simulink model "PositionComplementary"  (Simulink 6.6)
settings: Solver=ode4  StartTime=0.0  StopTime=60  FixedStep=SampleT  RelTol=1e-3
InitFcn:
  | clc
  | Taxi_Var_new
  | failures
  | insInit
  | piccolo_init
values from neighbouring files (symbols this model uses):
  A1 = 0    [Taxi_Var.m]    (also in Taxi_Var_new.m = 0.007)
  Apolar = 0.0899    [Taxi_Var.m]    (also in Taxi_Var_new.m = 0.057)
  CD0 = 0.0219    [Taxi_Var.m]    (also in Taxi_Var_new.m = 0.022)
  chord = S/span    (= 0.384036716878)    [Taxi_Var.m]    (also in Taxi_Var_new.m = 0.351341681574)
  CL0 = 0.1857    [Taxi_Var.m]    (also in Taxi_Var_new.m = 0.38)
  CLa = 4.6206    [Taxi_Var.m]    (also in Taxi_Var_new.m = 18.5)
  CLa_dot = 1.93    [Taxi_Var.m]    (also in Taxi_Var_new.m = 2.64)
  Clb = -0.0043    [Taxi_Var.m]    (also in Taxi_Var_new.m = -0.06)
  ClDa = 0.1695    [Taxi_Var.m]    (also in Taxi_Var_new.m)
  CLDe = 0.4032    [Taxi_Var.m]    (also in Taxi_Var_new.m = 0.24)
  CLDf = 0.047    [Taxi_Var.m]    (also in Taxi_Var_new.m = 0.4)
  ClDr = 0.0003    [Taxi_Var.m]    (also in Taxi_Var_new.m = 0.055)
  Clp = -0.4425    [Taxi_Var.m]    (also in Taxi_Var_new.m = -0.88)
  CLq = 8.7465    [Taxi_Var.m]    (also in Taxi_Var_new.m = 7.4)
  Clr = 0.0675    [Taxi_Var.m]    (also in Taxi_Var_new.m = 0.04)
  Cm0 = -0.0902    [Taxi_Var.m]    (also in Taxi_Var_new.m = 0.56)
  Cma = -1.3995    [Taxi_Var.m]    (also in Taxi_Var_new.m = -1.58)
  CmDe = -0.9493    [Taxi_Var.m]    (also in Taxi_Var_new.m = -41)
  CmDf = -.021    (= -0.021)    [Taxi_Var.m]    (also in Taxi_Var_new.m)
  Cmq = -10.8760    (= -10.876)    [Taxi_Var.m]    (also in Taxi_Var_new.m = -12)
  Cnb = 0.0281    [Taxi_Var.m]    (also in Taxi_Var_new.m = 0.73)
  CnDa = -0.0031    [Taxi_Var.m]    (also in Taxi_Var_new.m = -0.032)
  CnDr = -0.0882    [Taxi_Var.m]    (also in Taxi_Var_new.m = 0.19)
  Cnp = -0.0695    [Taxi_Var.m]    (also in Taxi_Var_new.m = -0.1)
  Cnr = -0.1045    [Taxi_Var.m]    (also in Taxi_Var_new.m = -0.23)
  CYb = -0.1999    [Taxi_Var.m]    (also in Taxi_Var_new.m = -0.98)
  CYDr = 0.0192    [Taxi_Var.m]    (also in Taxi_Var_new.m = 0.066)
  damax = 25*deg2rad    (= 0.436332312999)    [Taxi_Var.m]    (also in piccolo_init.m)
  damin = -25*deg2rad    (= -0.436332312999)    [Taxi_Var.m]    (also in piccolo_init.m)
  datrim = 0*deg2rad    (= 0)    [Taxi_Var.m]    (also in piccolo_init.m)
  demax = 15*deg2rad    (= 0.261799387799)    [Taxi_Var.m]    (also in piccolo_init.m)
  demin = -15*deg2rad    (= -0.261799387799)    [Taxi_Var.m]    (also in piccolo_init.m)
  detrim = -2.4137*deg2rad    (= -0.0421270121554)    [Taxi_Var.m]    (also in piccolo_init.m = -0.0523598775598)
  dfland = 30*deg2rad    (= 0.523598775598)    [Taxi_Var.m]    (also in piccolo_init.m)
  dfmax = 30*deg2rad    (= 0.523598775598)    [Taxi_Var.m]    (also in piccolo_init.m)
  dfmin = 0*deg2rad    (= 0)    [Taxi_Var.m]    (also in piccolo_init.m)
  drmax = 25*deg2rad    (= 0.436332312999)    [Taxi_Var.m]    (also in piccolo_init.m)
  drmin = -25*deg2rad    (= -0.436332312999)    [Taxi_Var.m]    (also in piccolo_init.m)
  drtrim = 0*deg2rad    (= 0)    [Taxi_Var.m]    (also in piccolo_init.m)
  dtmax = 1    [Taxi_Var.m]    (also in piccolo_init.m = 0.7)
  dtmin = 0    [Taxi_Var.m]    (also in piccolo_init.m = 0.25)
  dttrim = 0.0725    [Taxi_Var.m]    (also in piccolo_init.m = 0.35)
  Euler_0 = [0; 0; 45]'*pi/180    [Taxi_Var.m]    (also in Taxi_Var_new.m = [0 0 45]'*pi/180)
  IdxCmdOrbitRadius = 17    [piccolo_init.m]
  IdxCmdOrbitSense = 18    [piccolo_init.m]
  IdxCmdWp1Alt = 13    [piccolo_init.m]
  IdxCmdWp1Lat = 11    [piccolo_init.m]
  IdxCmdWp1Lon = 12    [piccolo_init.m]
  IdxCmdWp2Alt = 16    [piccolo_init.m]
  IdxCmdWp2Lat = 14    [piccolo_init.m]
  IdxCmdWp2Lon = 15    [piccolo_init.m]
  IdxEstimReserved1 = 4    [piccolo_init.m]
  IdxEstimWEast = 3    [piccolo_init.m]
  IdxEstimWNorth = 2    [piccolo_init.m]
  IdxGainsAltD = 10    [piccolo_init.m]
  IdxGainsAltI = 9    [piccolo_init.m]
  IdxGainsAltP = 8    [piccolo_init.m]
  IdxGainsPdynD = 4    [piccolo_init.m]
  IdxGainsPdynI = 3    [piccolo_init.m]
  IdxGainsPdynP = 2    [piccolo_init.m]
  IdxGainsPitchD = 7    [piccolo_init.m]
  IdxGainsPitchI = 6    [piccolo_init.m]
  IdxGainsPitchP = 5    [piccolo_init.m]
  IdxGainsRollD = 17    [piccolo_init.m]
  IdxGainsRollI = 16    [piccolo_init.m]
  IdxGainsRollP = 15    [piccolo_init.m]
  IdxGainsSlopeElevatorD = 25    [piccolo_init.m]
  IdxGainsSlopeElevatorP = 26    [piccolo_init.m]
  IdxGainsTrackConv = 24    [piccolo_init.m]
  IdxGainsTrackD = 23    [piccolo_init.m]
  IdxGainsTrackI = 22    [piccolo_init.m]
  IdxGainsTrackP = 21    [piccolo_init.m]
  IdxGainsTurnD = 14    [piccolo_init.m]
  IdxGainsTurnI = 13    [piccolo_init.m]
  IdxGainsTurnP = 12    [piccolo_init.m]
  IdxGainsYawD = 20    [piccolo_init.m]
  IdxGainsYawI = 19    [piccolo_init.m]
  IdxGainsYawP = 18    [piccolo_init.m]
  IdxLimitsAileronMax = 11    [piccolo_init.m]
  IdxLimitsAileronMin = 10    [piccolo_init.m]
  IdxLimitsBankMax = 9    [piccolo_init.m]
  IdxLimitsBankMin = 8    [piccolo_init.m]
  IdxLimitsElevatorMax = 13    [piccolo_init.m]
  IdxLimitsElevatorMin = 12    [piccolo_init.m]
  IdxLimitsFlapMax = 19    [piccolo_init.m]
  IdxLimitsFlapMin = 18    [piccolo_init.m]
  IdxLimitsPdynMax = 3    [piccolo_init.m]
  IdxLimitsPdynMin = 2    [piccolo_init.m]
  IdxLimitsRudderMax = 15    [piccolo_init.m]
  IdxLimitsRudderMin = 14    [piccolo_init.m]
  IdxLimitsThrottleMax = 17    [piccolo_init.m]
  IdxLimitsThrottleMin = 16    [piccolo_init.m]
  IdxSensorsAlt = 5    [piccolo_init.m]
  IdxSensorsLat = 3    [piccolo_init.m]
  IdxSensorsLon = 4    [piccolo_init.m]
  IdxSensorsVDown = 8    [piccolo_init.m]
  IdxSensorsVEast = 7    [piccolo_init.m]
  IdxSensorsVNorth = 6    [piccolo_init.m]
  IdxStatesGlobal = 2    [piccolo_init.m]
  IdxStatesManual = 16    [piccolo_init.m]
  IdxStatesMode = 15    [piccolo_init.m]
  ISA_g = 9.815    [Taxi_Var.m]    (also in Taxi_Var_new.m)
  ISA_hmax = 2000    [Taxi_Var.m]    (also in Taxi_Var_new.m)
  ISA_lapse = .0065    (= 0.0065)    [Taxi_Var.m]    (also in Taxi_Var_new.m)
  ISA_P0 = 101325    [Taxi_Var.m]    (also in Taxi_Var_new.m)
  ISA_R = 287    [Taxi_Var.m]    (also in Taxi_Var_new.m)
  ISA_rho0 = 1.225    [Taxi_Var.m]    (also in Taxi_Var_new.m)
  ISA_T0 = 289    [Taxi_Var.m]    (also in Taxi_Var_new.m)
  Ixx = 3.689084    [Taxi_Var.m]    (also in Taxi_Var_new.m = 3.8)
  Iyy = 7.43789    [Taxi_Var.m]    (also in Taxi_Var_new.m = 9.58)
  Izz = 10.22202    [Taxi_Var.m]    (also in Taxi_Var_new.m = 9.68)
  mass = 22.5    [Taxi_Var.m]    (also in Taxi_Var_new.m = 8.16466266)
  MinThK = 0.075    [Taxi_Var.m]    (also in Taxi_Var_new.m = 0.077)
  Pos_0 = [0; 0; 1000]'    [Taxi_Var.m]    (also in Taxi_Var_new.m = [0 0 500]')
  PQR_0 = [0; 0; 0]'    [Taxi_Var.m]    (also in Taxi_Var_new.m = [ 0 0 0]'*pi/180)
  SampleT = 0.005    [failures.m]
  span = 2.3368    [Taxi_Var.m]    (also in Taxi_Var_new.m = 2.795)
  TFact = 0.4    [Taxi_Var.m]    (also in Taxi_Var_new.m)
  ThK = 2.18    [Taxi_Var.m]    (also in Taxi_Var_new.m = 2.17)
  tsamp = APtsamp    (= 0.05)    [piccolo_init.m]
  ... (+1 more)
undefined symbols (not defined in the file or in its folder): clock, Earth, gaind, polesd, WGS84, zerosd
libraries: piccolo_library x60, simulink x45, aerolibconvert2 x13, dspsigops x5, aerolibasang x5, aerolibatmos2 x2, aerolibtransform2 x2, aerolibnav x2, aerolibutil x1, dspmtrx3 x1
(part 1 of 5)
CloseFcn:
  | rtwprivate ssgencode ModelCloseRequest AttitudeComplementary
settings Model: Creator=ASL_Lab  LastModifiedBy=ASL_Lab
settings DebuggingCC: MultiTaskDSMMsg=warning  MultiTaskCondExecSysMsg=none  StrictBusMsg=None
settings HardwareCC: TargetHWDeviceType=32-bit Generic
settings RTWCC: IncludeERTFirstTime=on

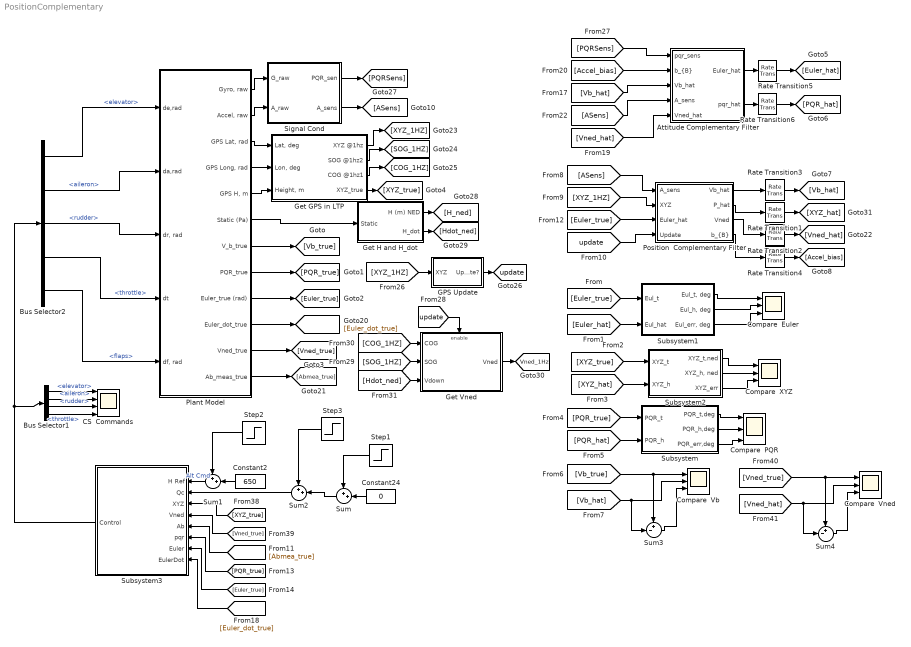
== system PositionComplementary ==
  Attitude Complementary Filter : Subsystem  mask{K1=25, K2=0.1, T=0.01, P0=Euler_0}
      mask prompts: K1 "Euler Gain K1"; K2 "Bias Gain K2"; T "Filter Execution Time"; P0 "Initial Euler"
      mask help: Attitude Complementary filter based on the Magneto-Pendular Sensor by Vasconcelos, et.al.
      mask Help: Help
  Bus Selector1 : BusSelector  OutputSignals=elevator,aileron,rudder,throttle
  Bus Selector2 : BusSelector  OutputSignals=elevator,aileron,rudder,throttle,flaps
  CS  Commands : Scope  NumInputPorts=4
      settings: TimeRange=44  YMin=0.0142~-2.5e-018~-1e-017~0.665  YMax=0.014425~2e-018~1e-017~0.735  SaveName=ScopeData19
  Compare  Euler : Scope  NumInputPorts=3
      settings: TimeRange=60  YMin=-20~-25.33803644914775~-0.3641680926328546  YMax=120~112.0265390106658~0.313830848443414  SaveName=ScopeData20
  Compare  PQR : Scope  NumInputPorts=3
      settings: TimeRange=200  YMin=-50~-350000~-450000  YMax=55~450000~350000  SaveName=ScopeData8
  Compare  Vb : Scope  NumInputPorts=3
      settings: TimeRange=44  YMin=-2.5~-800~-400  YMax=35~400~800  SaveName=ScopeData12
  Compare  Vned : Scope  NumInputPorts=3
      settings: TimeRange=44  YMin=-2.5~-800~-400  YMax=35~400~800  SaveName=ScopeData24
  Compare  XYZ : Scope  NumInputPorts=3
      settings: TimeRange=45  YMin=-800~-200~-32.89473684210498  YMax=800~1200~32.89473684210498  SaveName=ScopeData2
  Constant2 : Constant  Orientation=left  Value=650
  Constant24 : Constant  Orientation=left  Value=0
  GPS Update : Subsystem
  Get GPS in LTP : Subsystem
  "Get H and H_dot " : Subsystem
  Get Vned : Subsystem
  Plant Model : Subsystem
  Position  Complementary Filter : Subsystem  mask{K1=50, K2=75, K3=0.1, T=0.01, P0=Pos_0}
      mask prompts: K1 "Position Gain K1"; K2 "Velocity Gain K2"; K3 "Bias Gain K3"; T "Filter Execution Time"; P0 "Initial Position"
      mask help: Position Complementary filter based on the Magneto-Pendular Sensor by Vasconcelos, et.al.
      mask Help: Help
  Rate Transition{1..6} (6 alike) : RateTransition  OutPortSampleTime=0.005
  Signal Cond : Subsystem
  Step1 : Step  Orientation=left  Time=15  After=3*pi/180  SampleTime=0
  Step2 : Step  Orientation=left  Time=35  After=250  SampleTime=0
  Step3 : Step  Orientation=left  Time=35  After=-4*pi/180  SampleTime=0
  Subsystem : Subsystem
  Subsystem1 : Subsystem
  Subsystem2 : Subsystem
  Subsystem3 : Subsystem  Orientation=left
  Sum : Sum  Orientation=left  Inputs=++|  SaturateOnIntegerOverflow=on
  Sum1 : Sum  Orientation=left  Inputs=++|  SaturateOnIntegerOverflow=on
  Sum2 : Sum  Orientation=left  Inputs=++|  SaturateOnIntegerOverflow=on
  Sum3 : Sum  Inputs=+-|
  Sum4 : Sum  Inputs=+-|
  tag scope: Vned_1Hz=global, update=global
  wires:
  Plant Model/1("Gyro, raw") -> Signal Cond/1(G_raw)
  Plant Model/2("Accel, raw") -> Signal Cond/2(A_raw)
  Plant Model/3("GPS Lat, rad") -> Get GPS in LTP/1("Lat, deg")
  Plant Model/5("GPS H, m") -> Get GPS in LTP/3("Height, m")
  Plant Model/4("GPS Long, rad") -> Get GPS in LTP/2("Lon, deg")
  Plant Model/7(V_b_true) -> [Vb_true]
  Plant Model/8(PQR_true) -> [PQR_true]
  Plant Model/9(Euler_true (rad)) -> [Euler_true]
  Plant Model/11(Vned_true) -> [Vned_true]
  Subsystem1/1("Eul_t, deg") -> Compare  Euler/1
  Subsystem1/2("Eul_h, deg") -> Compare  Euler/2
  Subsystem1/3("Eul_err, deg") -> Compare  Euler/3
  [XYZ_true] -> Subsystem2/1(XYZ_t)
  [XYZ_hat] -> Subsystem2/2(XYZ_h)
  Subsystem/1(PQR_t,deg) -> Compare  PQR/1
  Subsystem/2(PQR_h,deg) -> Compare  PQR/2
  Subsystem/3(PQR_err,deg) -> Compare  PQR/3
  [Vb_true] -> Compare  Vb/1, Sum3/1
  [Vb_hat] -> Sum3/2, Compare  Vb/2
  Sum3/1 -> Compare  Vb/3
  Get GPS in LTP/4(XYZ_true) -> [XYZ_true]
  [PQR_true] -> Subsystem/1(PQR_t)
  [PQR_hat] -> Subsystem/2(PQR_h)
  [Euler_true] -> Subsystem1/1(Eul_t)
  [Euler_hat] -> Subsystem1/2(Eul_hat)
  Subsystem2/1(XYZ_t,ned) -> Compare  XYZ/1
  Subsystem2/2("XYZ_h, ned") -> Compare  XYZ/2
  Subsystem2/3(XYZ_err) -> Compare  XYZ/3
  Constant24/1 -> Sum/2
  Step1/1 -> Sum/1
  Constant2/1 -> Sum1/2
  Step2/1 -> Sum1/1
  Plant Model/10(Euler_dot_true) -> [Euler_dot_true]
  Plant Model/12(Ab_meas_true) -> [Abmea_true]
  Plant Model/6(Static (Pa)) -> "Get H and H_dot "/1(Static)
  Signal Cond/2(A_sens) -> [ASens]
  Get GPS in LTP/1(XYZ @1hz) -> [XYZ_1HZ]
  Get GPS in LTP/2(SOG @1hz2) -> [SOG_1HZ]
  Get GPS in LTP/3(COG @1hz1) -> [COG_1HZ]
  GPS Update/1(Update?) -> [update]
  [XYZ_1HZ] -> GPS Update/1(XYZ)
  Signal Cond/1(PQR_sen) -> [PQRSens]
  [update] -> Get Vned/Enable
  [COG_1HZ] -> Get Vned/1(COG)
  [SOG_1HZ] -> Get Vned/2(SOG)
  "Get H and H_dot "/1(H (m) NED) -> [H_ned]
  "Get H and H_dot "/2(H_dot) -> [Hdot_ned]
  [Hdot_ned] -> Get Vned/3(Vdown)
  Get Vned/1(Vned) -> [Vned_1Hz]
  Sum1/1 -> Subsystem3/1(H Ref)  "Alt Cmd"
  [ASens] -> Position  Complementary Filter/1(A_sens)
  [XYZ_1HZ] -> Position  Complementary Filter/2(XYZ)
  [Euler_true] -> Position  Complementary Filter/3(Euler_hat)
  [update] -> Position  Complementary Filter/4(Update)
  Position  Complementary Filter/1(Vb_hat) -> Rate Transition3/1
  Position  Complementary Filter/2(P_hat) -> Rate Transition1/1
  [XYZ_true] -> Subsystem3/3(XYZ)
  [Vned_true] -> Subsystem3/4(Vned)
  [Abmea_true] -> Subsystem3/5(Ab)
  [PQR_true] -> Subsystem3/6(pqr)
  [Euler_true] -> Subsystem3/7(Euler)
  [Euler_dot_true] -> Subsystem3/8(EulerDot)
  Subsystem3/1(Control) -> Bus Selector2/1, Bus Selector1/1
  Bus Selector2/1 -> Plant Model/1(de,rad)  "<elevator>"
  Bus Selector2/2 -> Plant Model/2(da,rad)  "<aileron>"
  Bus Selector2/3 -> Plant Model/3("dr, rad")  "<rudder>"
  Bus Selector2/4 -> Plant Model/4(dt)  "<throttle>"
  Bus Selector2/5 -> Plant Model/5("df, rad")  "<flaps>"
  Rate Transition3/1 -> [Vb_hat]
  Rate Transition1/1 -> [XYZ_hat]
  Bus Selector1/1 -> CS  Commands/1  "<elevator>"
  Bus Selector1/2 -> CS  Commands/2  "<aileron>"
  Bus Selector1/3 -> CS  Commands/3  "<rudder>"
  Bus Selector1/4 -> CS  Commands/4  "<throttle>"
  Sum2/1 -> Subsystem3/2(Qc)
  Sum/1 -> Sum2/2
  Step3/1 -> Sum2/1
  Rate Transition2/1 -> [Vned_hat]
  Position  Complementary Filter/3(Vned) -> Rate Transition2/1
  [Vned_true] -> Sum4/1, Compare  Vned/1
  [Vned_hat] -> Compare  Vned/2, Sum4/2
  Sum4/1 -> Compare  Vned/3
  Position  Complementary Filter/4("b_{B}") -> Rate Transition4/1
  Rate Transition4/1 -> [Accel_bias]
  [PQRSens] -> Attitude Complementary Filter/1(pqr_sens)
  Attitude Complementary Filter/1(Euler_hat) -> Rate Transition5/1
  Attitude Complementary Filter/2(pqr_hat) -> Rate Transition6/1
  [ASens] -> Attitude Complementary Filter/4(A_sens)
  [Accel_bias] -> Attitude Complementary Filter/2("b_{B}")
  [Vb_hat] -> Attitude Complementary Filter/3(Vb_hat)
  [Vned_hat] -> Attitude Complementary Filter/5(Vned_hat)
  Rate Transition5/1 -> [Euler_hat]
  Rate Transition6/1 -> [PQR_hat]

== system PositionComplementary/Attitude Complementary Filter ==
  pqr_sens : Inport
  "b_{B}" : Inport  Port=2
  Vb_hat : Inport  Port=3
  A_sens : Inport  Port=4
  Vned_hat : Inport  Port=5
  Embedded MATLAB Function : Stateflow chart
  Embedded MATLAB Function1 : Stateflow chart
  IC : InitialCondition  Value=P0  SampleTime=T
  Integer Delay4 : simulink/Discrete/Integer Delay  Orientation=left  vinit=0.0  samptime=-1  NumDelays=1
  Integer Delay5 : simulink/Discrete/Integer Delay  Orientation=left  vinit=0.0  samptime=-1  NumDelays=1
  K1 : Gain  Orientation=left  Gain=K1
  K2 : Gain  Orientation=left  Gain=K2
  Subsystem : Subsystem
  Sum5 : Sum  Orientation=down  Inputs=-+|
  Sum6 : Sum  Inputs=|++
  Sum8 : Sum  Inputs=4
  T3 : Gain  Gain=T
  T4 : Gain  Gain=T
  inertial to body : Stateflow chart
  Euler_hat : Outport  Orientation=left
  pqr_hat : Outport  Orientation=left  Port=2
  wires:
  Embedded MATLAB Function/1(euler_dot) -> T3/1
  Subsystem/1(Euler) -> [Euler], Embedded MATLAB Function/1(euler)
  T3/1 -> Sum8/1
  Subsystem/2(pqr_nb) -> Embedded MATLAB Function/2(pqr), pqr_hat/1
  Sum8/1 -> Integer Delay4/1, Euler_hat/1, IC/1
  [Euler] -> Sum5/2
  Integer Delay4/1 -> Sum8/4
  K1/1 -> Sum8/3
  inertial to body/1(pqr) -> Sum6/1
  Sum6/1 -> Embedded MATLAB Function1/2(pqr), Integer Delay5/1, [bg_b]
  [Euler] -> Embedded MATLAB Function1/1(euler)
  [Euler] -> inertial to body/1(euler)
  Embedded MATLAB Function1/1(euler_dot) -> T4/1
  T4/1 -> Sum8/2
  Integer Delay5/1 -> Sum6/2
  K2/1 -> inertial to body/2(euler_dot)
  [bg_b] -> Subsystem/1("bg_{B}")
  pqr_sens/1 -> Subsystem/2(pqr_sens)
  "b_{B}"/1 -> Subsystem/3("b_{B}")
  Vb_hat/1 -> Subsystem/4(Vb_hat)
  A_sens/1 -> Subsystem/5(A_sens)
  Vned_hat/1 -> Subsystem/6(Vned_hat)
  Sum5/1 -> K1/1, K2/1
  IC/1 -> Sum5/1

== system PositionComplementary/GPS Update ==
  XYZ : Inport
  Demux : Demux  Outputs=3
  Detect Change : Subsystem
  Detect Change1 : Subsystem
  Detect Change2 : Subsystem
  Saturation1 : Saturate  UpperLimit=1  LowerLimit=0  SampleTime=SampleT
  Sum : Sum  Inputs=3
  Update? : Outport
  wires:
  Demux/1 -> Detect Change/1(Data)
  Demux/2 -> Detect Change1/1(Data)
  Demux/3 -> Detect Change2/1(Data)
  Detect Change/1(change?) -> Sum/1
  Detect Change1/1(change?) -> Sum/2
  Detect Change2/1(change?) -> Sum/3
  Sum/1 -> Saturation1/1
  XYZ/1 -> Demux/1
  Saturation1/1 -> Update?/1

== system PositionComplementary/Get GPS in LTP ==
  "Lat, deg" : Inport
  "Lon, deg" : Inport  Port=2
  "Height, m" : Inport  Port=3
  Angle Conversion1 : aerolibconvert2/Angle Conversion  SystemSampleTime=-1  IU=rad  OU=deg
  Angle Conversion2 : aerolibconvert2/Angle Conversion  SystemSampleTime=-1  IU=rad  OU=deg
  Constant : Constant  Orientation=left  Value=[0 , 37.0004768371582, -122.061897277832]
  Demux : Demux  Outputs=3
  Demux1 : Demux  Outputs=3
  Discrete Derivative : simulink/Discrete/Discrete Derivative  SystemSampleTime=-1  gainval=1.0  ICPrevScaledInput=0.0  OutDataType=sfix(16)  OutScaling=2^-10  DoSatur=off
  Embedded MATLAB Function1 : Stateflow chart
  Fcn : Fcn  Expr=sqrt(u(1)^2+u(2)^2+u(3)^2)
  Geod2LTP2 : Subsystem
      mask Description:
      | This block provides transformation of the Geodetic coordinates
      | to the LTP coorinate system. The block uses two consecutive transformations
      | (Geodetic -> ECEF ->LTP).
      | Geodetic coordinates of the LTP origin should also be predetermined.
      mask Help: Oops!
      mask Display: plot(0,0,100,100,[45,40,35,40,40],[85,95,85,95,40],[85,95,85,95,40],[35,40,45,40,40],[60,40,10,20,10,14],[70,40,10,13,10,20],[56,45],[70,70],[60,60],[50,60],[60,60],[30,40],[50,60],[20,20],[30,40],[20,20],[45,55],[35,25],[75,65],[35,25])
  Mux : Mux  Inputs=3
  NEU2NED : Gain  Gain=[1 0 0;0 1 0;0 0 -1]  Multiplication=Matrix(K*u)  SaturateOnIntegerOverflow=on
  NEU2NED1 : Gain  Gain=[1 0 0;0 1 0;0 0 -1]  Multiplication=Matrix(K*u)  SaturateOnIntegerOverflow=on
  Reshape1 : Reshape
  Sim Latency : Subsystem
  Sim Latency3 : Subsystem
  Sim Latency4 : Subsystem
  Sim Latency5 : Subsystem
  Sim Latency6 : Subsystem
  XYZ @1hz : Outport
  SOG @1hz2 : Outport  Port=2
  COG @1hz1 : Outport  Port=3
  XYZ_true : Outport  Port=4
  wires:
  Constant/1 -> Geod2LTP2/1("Height, Lat, Lon Initials from GPS")
  Geod2LTP2/1("NEU, m") -> Demux1/1, Discrete Derivative/1, Reshape1/1
  "Lat, deg"/1 -> Angle Conversion1/1
  "Lon, deg"/1 -> Angle Conversion2/1
  "Height, m"/1 -> Geod2LTP2/4(Hight,m(GPS))
  Fcn/1 -> Sim Latency6/1(Fast Data)
  Embedded MATLAB Function1/1(cog) -> Sim Latency5/1(Fast Data)
  Discrete Derivative/1 -> Demux/1, Fcn/1
  Mux/1 -> NEU2NED1/1
  Angle Conversion1/1 -> Geod2LTP2/2("Lat, deg(GPS)")
  Angle Conversion2/1 -> Geod2LTP2/3("Lon, deg(GPS)")
  Demux1/1 -> Sim Latency/1(Fast Data)
  Demux1/2 -> Sim Latency3/1(Fast Data)
  Demux1/3 -> Sim Latency4/1(Fast Data)
  Sim Latency/1(1Hz Data) -> Mux/1
  Sim Latency3/1(1Hz Data) -> Mux/2
  Sim Latency4/1(1Hz Data) -> Mux/3
  Sim Latency5/1(1Hz Data) -> COG @1hz1/1
  Sim Latency6/1(1Hz Data) -> SOG @1hz2/1
  Reshape1/1 -> NEU2NED/1
  NEU2NED/1 -> XYZ_true/1
  Demux/1 -> Embedded MATLAB Function1/1(Vn)
  Demux/2 -> Embedded MATLAB Function1/2(Ve)
  NEU2NED1/1 -> XYZ @1hz/1

== system PositionComplementary/Get H and H_dot  ==
  Static : Inport
  Discrete Derivative : simulink/Discrete/Discrete Derivative  SystemSampleTime=-1  gainval=1.0  ICPrevScaledInput=-0.6  OutDataType=sfix(16)  OutScaling=2^-10  DoSatur=off
  Gain : Gain  Gain=-1
  Pressure Altitude : aerolibatmos2/Pressure Altitude  SystemSampleTime=-1  units=Metric (MKS)  action=Warning
  H (m) NED : Outport
  H_dot : Outport  Port=2
  wires:
  Pressure Altitude/1 -> Gain/1
  Gain/1 -> Discrete Derivative/1, H (m) NED/1
  Discrete Derivative/1 -> H_dot/1
  Static/1 -> Pressure Altitude/1

== system PositionComplementary/Get Vned ==
  COG : Inport
  SOG : Inport  Port=2
  Vdown : Inport  Port=3
  Enable : EnablePort
  Embedded MATLAB Function1 : Stateflow chart
  Mux1 : Mux  Inputs=3
  Vned : Outport
  wires:
  Embedded MATLAB Function1/1(Vn) -> Mux1/1
  Embedded MATLAB Function1/2(Ve) -> Mux1/2
  Vdown/1 -> Mux1/3
  Mux1/1 -> Vned/1
  COG/1 -> Embedded MATLAB Function1/2(cog)
  SOG/1 -> Embedded MATLAB Function1/1(sog)

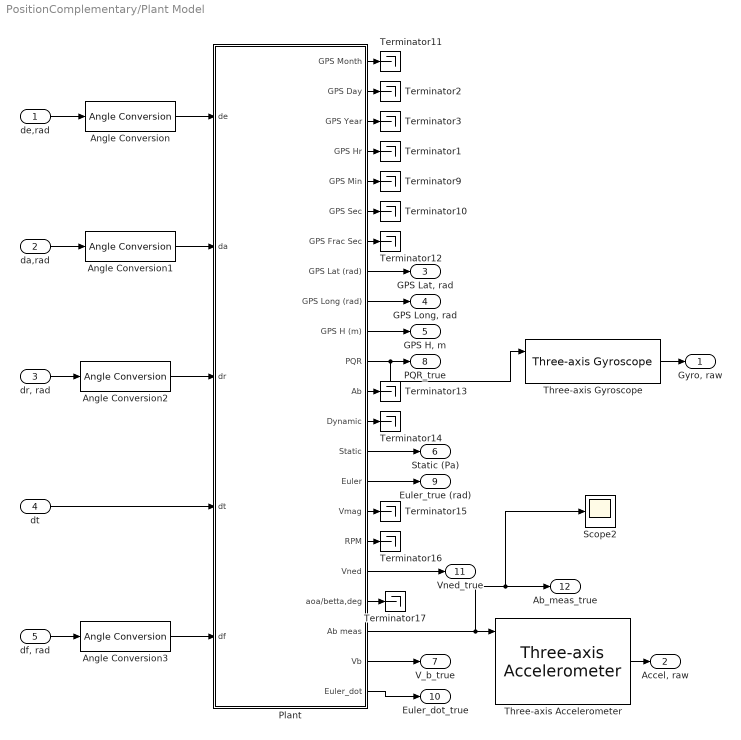
== system PositionComplementary/Plant Model ==
  de,rad : Inport
  da,rad : Inport  Port=2
  "dr, rad" : Inport  Port=3
  dt : Inport  Port=4
  "df, rad" : Inport  Port=5
  Angle Conversion{,1..3} (4 alike) : aerolibconvert2/Angle Conversion  SystemSampleTime=-1  IU=rad  OU=deg
  Plant : Subsystem
  Scope2 : Scope
      settings: TimeRange=44  YMin=-45  YMax=20  SaveName=ScopeData33
  Terminator{1..3,9..17} (12 alike) : Terminator
  Three-axis Accelerometer : aerolibnav/Three-axis Accelerometer  SystemSampleTime=-1  units=Metric (MKS)  acc=[0 0 0]  gtype=off  dtype_a=on  w_a=190  z_a=0.707  a_sf_cc=[-41 0 0; 0 41 0; 0 0 -43]  a_bias=[2015 2018 2006]  a_rand=on  a_seeds=[23093 23094 23095]  a_pow=[0.008 0.008 0.008]  a_sat="[-inf  -inf  -inf  inf inf inf]"  a_Ts=SampleT
  Three-axis Gyroscope : aerolibnav/Three-axis Gyroscope  SystemSampleTime=-1  dtype_g=on  w_g=190  z_g=0.707  g_sf_cc=[-142 0 0; 0 142 0; 0 0 235]  g_bias=[1866 1981 2042]  g_sen=[0 0 0]  g_rand=on  g_seeds=[23093 23094 23095]  g_pow=[0.008 0.008 0.008]  g_sat="[-inf  -inf  -inf  inf inf inf]"  g_Ts=SampleT
  "Gyro, raw" : Outport
  "Accel, raw" : Outport  Port=2
  "GPS Lat, rad" : Outport  Port=3
  "GPS Long, rad" : Outport  Port=4
  "GPS H, m" : Outport  Port=5
  Static (Pa) : Outport  Port=6
  V_b_true : Outport  Port=7
  PQR_true : Outport  Port=8
  Euler_true (rad) : Outport  Port=9
  Euler_dot_true : Outport  Port=10
  Vned_true : Outport  Port=11
  Ab_meas_true : Outport  Port=12
  wires:
  Three-axis Gyroscope/1 -> "Gyro, raw"/1
  Three-axis Accelerometer/1 -> "Accel, raw"/1
  Plant/11(PQR) -> PQR_true/1, Three-axis Gyroscope/1
  Plant/14(Static) -> Static (Pa)/1
  Plant/8(GPS Lat (rad)) -> "GPS Lat, rad"/1
  Plant/9(GPS Long (rad)) -> "GPS Long, rad"/1
  Plant/10(GPS H (m)) -> "GPS H, m"/1
  Plant/20(Ab meas) -> Three-axis Accelerometer/1, Ab_meas_true/1, Scope2/1
  Plant/21(Vb) -> V_b_true/1
  Plant/15(Euler) -> Euler_true (rad)/1
  Plant/18(Vned) -> Vned_true/1
  Plant/1(GPS Month) -> Terminator11/1
  Plant/2(GPS Day) -> Terminator2/1
  Plant/3(GPS Year) -> Terminator3/1
  Plant/4(GPS Hr) -> Terminator1/1
  Plant/5(GPS Min) -> Terminator9/1
  Plant/6(GPS Sec) -> Terminator10/1
  Plant/7(GPS Frac Sec) -> Terminator12/1
  Plant/12(Ab) -> Terminator13/1
  Plant/13(Dynamic) -> Terminator14/1
  Plant/16(Vmag) -> Terminator15/1
  Plant/17(RPM) -> Terminator16/1
  Plant/19(aoa/betta,deg) -> Terminator17/1
  de,rad/1 -> Angle Conversion/1
  da,rad/1 -> Angle Conversion1/1
  "dr, rad"/1 -> Angle Conversion2/1
  dt/1 -> Plant/4(dt)
  "df, rad"/1 -> Angle Conversion3/1
  Angle Conversion/1 -> Plant/1(de)
  Angle Conversion1/1 -> Plant/2(da)
  Angle Conversion2/1 -> Plant/3(dr)
  Angle Conversion3/1 -> Plant/5(df)
  Plant/22(Euler_dot) -> Euler_dot_true/1

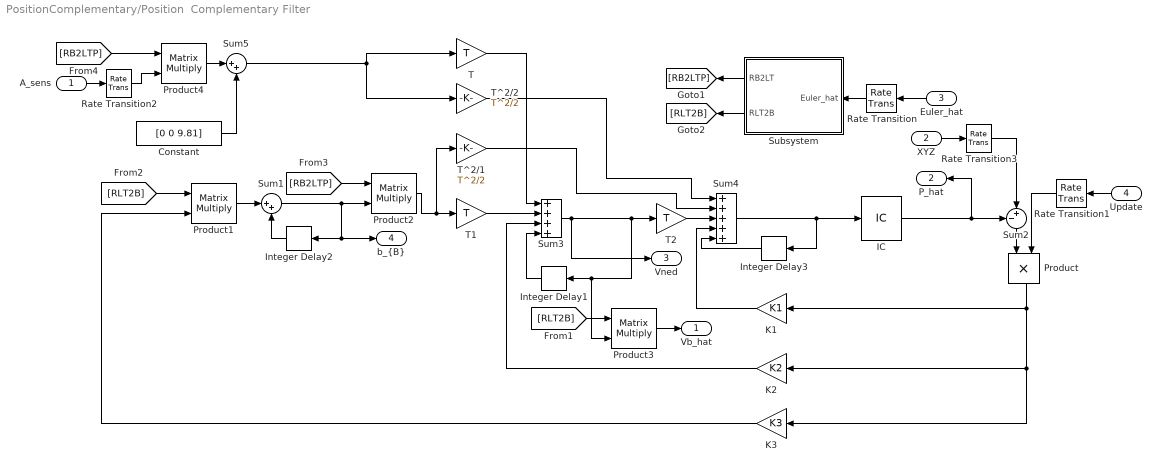
== system PositionComplementary/Position  Complementary Filter ==
  A_sens : Inport
  XYZ : Inport  Port=2
  Euler_hat : Inport  Orientation=left  Port=3
  Update : Inport  Orientation=left  Port=4
  Constant : Constant  Value=[0 0 9.81]  SampleTime=0.01
  IC : InitialCondition  Value=P0  SampleTime=T
  Integer Delay1 : simulink/Discrete/Integer Delay  Orientation=left  vinit=0.0  samptime=-1  NumDelays=1
  Integer Delay2 : simulink/Discrete/Integer Delay  Orientation=left  vinit=0.0  samptime=-1  NumDelays=1
  Integer Delay3 : simulink/Discrete/Integer Delay  Orientation=left  vinit=0.0  samptime=-1  NumDelays=1
  K1 : Gain  Orientation=left  Gain=K1
  K2 : Gain  Orientation=left  Gain=K2
  K3 : Gain  Orientation=left  Gain=K3
  Product : Product  Orientation=down  RndMeth=Zero
  Product{1..4} (4 alike) : Product  Multiplication=Matrix(*)  RndMeth=Zero
  Rate Transition : RateTransition  Orientation=left  OutPortSampleTime=T
  Rate Transition1 : RateTransition  Orientation=left  OutPortSampleTime=T
  Rate Transition2 : RateTransition  OutPortSampleTime=T
  Rate Transition3 : RateTransition  OutPortSampleTime=T
  Subsystem : Subsystem  Orientation=left
  Sum1 : Sum  Inputs=|++
  Sum2 : Sum  Orientation=down  Inputs=-+|
  Sum3 : Sum  Inputs=4
  Sum4 : Sum  Inputs=5
  Sum5 : Sum  Inputs=|++
  T : Gain  Gain=T
  T1 : Gain  Gain=T
  T2 : Gain  Gain=T
  T^2/1 : Gain  Gain=T^2/2
  T^2/2 : Gain  Gain=T^2/2
  Vb_hat : Outport
  P_hat : Outport  Orientation=left  Port=2
  Vned : Outport  Port=3
  "b_{B}" : Outport  Port=4
  wires:
  Subsystem/2(RLT2B) -> [RLT2B]
  Subsystem/1(RB2LT) -> [RB2LTP]
  Euler_hat/1 -> Rate Transition/1
  K3/1 -> Product1/2
  Product1/1 -> Sum1/1
  Sum1/1 -> Product2/2, Integer Delay2/1, "b_{B}"/1
  Product2/1 -> T^2/1/1, T1/1
  T1/1 -> Sum3/2
  T/1 -> Sum3/1
  Sum3/1 -> T2/1, Integer Delay1/1, Product3/2, Vned/1
  K2/1 -> Sum3/3
  T2/1 -> Sum4/3
  T^2/1/1 -> Sum4/2
  T^2/2/1 -> Sum4/1
  Sum4/1 -> Integer Delay3/1, IC/1
  K1/1 -> Sum4/4
  XYZ/1 -> Rate Transition3/1
  Product3/1 -> Vb_hat/1
  Sum2/1 -> Product/1
  Product/1 -> K1/1, K2/1, K3/1
  Update/1 -> Rate Transition1/1
  Integer Delay3/1 -> Sum4/5
  Integer Delay2/1 -> Sum1/2
  Integer Delay1/1 -> Sum3/4
  A_sens/1 -> Rate Transition2/1
  Product4/1 -> Sum5/1
  Constant/1 -> Sum5/2
  Sum5/1 -> T/1, T^2/2/1
  Rate Transition/1 -> Subsystem/1(Euler_hat)
  Rate Transition1/1 -> Product/2
  Rate Transition3/1 -> Sum2/2
  [RLT2B] -> Product1/1
  [RB2LTP] -> Product4/1
  Rate Transition2/1 -> Product4/2
  [RB2LTP] -> Product2/1
  [RLT2B] -> Product3/1
  IC/1 -> Sum2/1, P_hat/1

== system PositionComplementary/Signal Cond ==
  G_raw : Inport
  A_raw : Inport  Port=2
  Accel Convert : Subsystem
  Gyro Convert : Subsystem
  PQR_sen : Outport
  A_sens : Outport  Port=2
  wires:
  G_raw/1 -> Gyro Convert/1(Raw)
  Gyro Convert/1(Comp) -> PQR_sen/1
  A_raw/1 -> Accel Convert/1(Raw)
  Accel Convert/1(Comp) -> A_sens/1

== system PositionComplementary/Subsystem ==
  PQR_t : Inport
  PQR_h : Inport  Port=2
  Angle Conversion1 : aerolibconvert2/Angle Conversion  SystemSampleTime=-1  IU=rad  OU=deg
  Angle Conversion5 : aerolibconvert2/Angle Conversion  SystemSampleTime=-1  IU=rad  OU=deg
  Angle Conversion6 : aerolibconvert2/Angle Conversion  SystemSampleTime=-1  IU=rad  OU=deg
  Sum2 : Sum  Inputs=+-|
  PQR_t,deg : Outport
  PQR_h,deg : Outport  Port=2
  PQR_err,deg : Outport  Port=3
  wires:
  PQR_t/1 -> Angle Conversion6/1, Sum2/1
  PQR_h/1 -> Angle Conversion1/1, Sum2/2
  Sum2/1 -> Angle Conversion5/1
  Angle Conversion6/1 -> PQR_t,deg/1
  Angle Conversion1/1 -> PQR_h,deg/1
  Angle Conversion5/1 -> PQR_err,deg/1

== system PositionComplementary/Subsystem1 ==
  Eul_t : Inport
  Eul_hat : Inport  Port=2
  Angle Conversion2 : aerolibconvert2/Angle Conversion  SystemSampleTime=-1  IU=rad  OU=deg
  Angle Conversion3 : aerolibconvert2/Angle Conversion  SystemSampleTime=-1  IU=rad  OU=deg
  Angle Conversion4 : aerolibconvert2/Angle Conversion  SystemSampleTime=-1  IU=rad  OU=deg
  Sum : Sum  Inputs=+-|
  "Eul_t, deg" : Outport
  "Eul_h, deg" : Outport  Port=2
  "Eul_err, deg" : Outport  Port=3
  wires:
  Eul_t/1 -> Sum/1, Angle Conversion4/1
  Eul_hat/1 -> Sum/2, Angle Conversion2/1
  Sum/1 -> Angle Conversion3/1
  Angle Conversion4/1 -> "Eul_t, deg"/1
  Angle Conversion2/1 -> "Eul_h, deg"/1
  Angle Conversion3/1 -> "Eul_err, deg"/1

== system PositionComplementary/Subsystem2 ==
  XYZ_t : Inport
  XYZ_h : Inport  Port=2
  Sum1 : Sum  Inputs=+-|
  XYZ_t,ned : Outport
  "XYZ_h, ned" : Outport  Port=2
  XYZ_err : Outport  Port=3
  wires:
  XYZ_h/1 -> Sum1/2, "XYZ_h, ned"/1
  XYZ_t/1 -> Sum1/1, XYZ_t,ned/1
  Sum1/1 -> XYZ_err/1

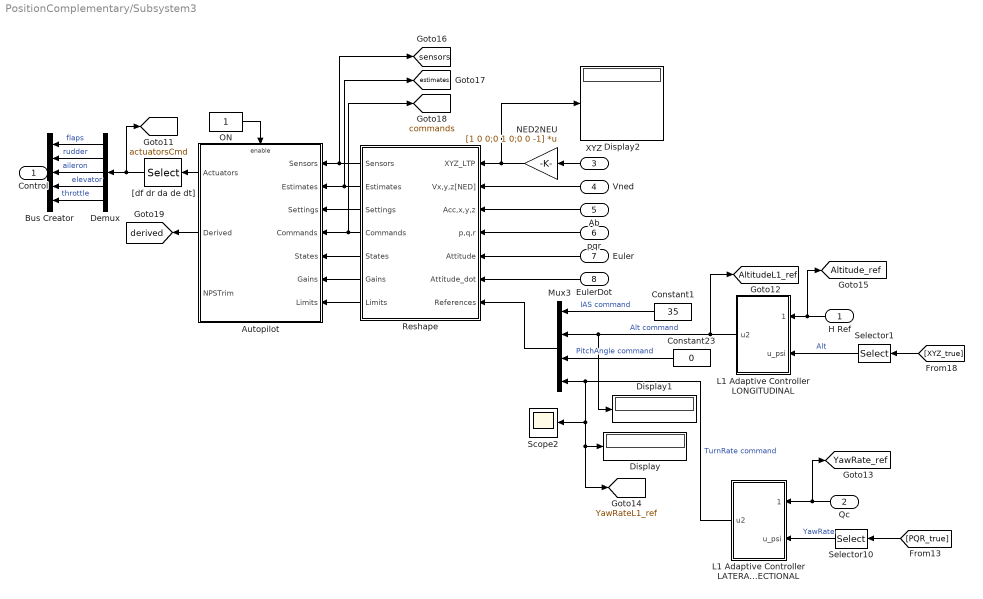
== system PositionComplementary/Subsystem3 ==
  H Ref : Inport  Orientation=left
  Qc : Inport  Orientation=left  Port=2
  XYZ : Inport  Orientation=left  Port=3
  Vned : Inport  Orientation=left  Port=4
  Ab : Inport  Orientation=left  Port=5
  pqr : Inport  Orientation=left  Port=6
  Euler : Inport  Orientation=left  Port=7
  EulerDot : Inport  Orientation=left  Port=8
  Autopilot : Subsystem  Orientation=left
  Bus Creator : BusCreator  Orientation=left  Inputs=5
  Constant1 : Constant  Orientation=left  Value=35
  Constant23 : Constant  Orientation=left  Value=0
  Demux : Demux  Orientation=left  Outputs=5
  Display : Display
  Display1 : Display
  Display2 : Display
  L1 Adaptive Controller LATERAL-DIRECTIONAL : Subsystem  Orientation=left  mask{gamma=-2000, m=4, omega=2, Pbound=.1, L1ONOFF=0}
      mask prompts: gamma "L1 gain"; m "state predictor (m)"; omega "low-pass filter (omega)"; Pbound "projection bounds"; L1ONOFF "L1 switch"
  L1 Adaptive Controller LONGITUDINAL : Subsystem  Orientation=left  mask{gamma=-1, m=4, omega=1, Pbound=50, L1ONOFF=0}
      mask prompts: gamma "L1 gain"; m "state predictor (m)"; omega "low-pass filter (omega)"; Pbound "projection bounds"; L1ONOFF "L1 switch"
  Mux3 : Mux  Orientation=left
  NED2NEU : Gain  Orientation=left  Gain=[1 0 0;0 1 0;0 0 -1]  Multiplication=Matrix(K*u)  SaturateOnIntegerOverflow=on
  ON : Constant
  Reshape : Subsystem  Orientation=left
  Scope2 : Scope
      settings: YMin=-1  YMax=1  SaveName=ScopeData29
  Selector1 : Selector  Orientation=left  IndexOptions=Index vector (dialog)  Indices=3  OutputSizes=1  InputPortWidth=3
  Selector10 : Selector  Orientation=left  IndexOptions=Index vector (dialog)  Indices=3  OutputSizes=1  InputPortWidth=3
  "[df dr da de dt]" : Selector  Orientation=left  IndexOptions=Index vector (dialog)  Indices=[10 6 2 4 8]  OutputSizes=[(-2)]  InputPortWidth=12
  Control : Outport  Orientation=left
  tag scope: AltitudeL1_ref=global, Altitude_ref=global, YawRateL1_ref=global, YawRate_ref=global, actuatorsCmd=global, commands=global, derived=global, estimates=global, sensors=global
  wires:
  XYZ/1 -> NED2NEU/1
  Vned/1 -> Reshape/2(Vx,y,z[NED])
  Ab/1 -> Reshape/3(Acc,x,y,z)
  pqr/1 -> Reshape/4(p,q,r)
  Reshape/1(Sensors) -> Autopilot/1(Sensors), [sensors]
  Reshape/2(Estimates) -> Autopilot/2(Estimates), [estimates]
  Reshape/3(Settings) -> Autopilot/3(Settings)
  Reshape/4(Commands) -> Autopilot/4(Commands), [commands]
  Reshape/5(States) -> Autopilot/5(States)
  Reshape/6(Gains) -> Autopilot/6(Gains)
  Reshape/7(Limits) -> Autopilot/7(Limits)
  ON/1 -> Autopilot/Enable
  Autopilot/1(Actuators) -> "[df dr da de dt]"/1
  "[df dr da de dt]"/1 -> Demux/1, [actuatorsCmd]
  Euler/1 -> Reshape/5(Attitude)
  EulerDot/1 -> Reshape/6(Attitude_dot)
  Autopilot/2(Derived) -> [derived]
  Constant1/1 -> Mux3/1  "IAS command"
  L1 Adaptive Controller LONGITUDINAL/1(u2) -> [AltitudeL1_ref], Mux3/2, Display1/1  "Alt command"
  Constant23/1 -> Mux3/3  "PitchAngle command"
  L1 Adaptive Controller LATERAL-DIRECTIONAL/1(u2) -> Mux3/4, Display/1, [YawRateL1_ref], Scope2/1  "TurnRate command"
  Mux3/1 -> Reshape/7(References)
  Qc/1 -> L1 Adaptive Controller LATERAL-DIRECTIONAL/1(u_psi_c), [YawRate_ref]
  [PQR_true] -> Selector10/1
  Selector10/1 -> L1 Adaptive Controller LATERAL-DIRECTIONAL/2(u_psi)  "YawRate"
  H Ref/1 -> L1 Adaptive Controller LONGITUDINAL/1(u_psi_c), [Altitude_ref]
  [XYZ_true] -> Selector1/1
  Selector1/1 -> L1 Adaptive Controller LONGITUDINAL/2(u_psi)  "Alt"
  Demux/1 -> Bus Creator/1  "flaps"
  Demux/2 -> Bus Creator/2  "rudder"
  Demux/3 -> Bus Creator/3  "aileron"
  Demux/4 -> Bus Creator/4  "elevator"
  Demux/5 -> Bus Creator/5  "throttle"
  NED2NEU/1 -> Reshape/1(XYZ_LTP), Display2/1
  Bus Creator/1 -> Control/1

== system PositionComplementary/Attitude Complementary Filter/Subsystem ==
  "bg_{B}" : Inport  Orientation=left
  pqr_sens : Inport  Port=2
  "b_{B}" : Inport  Port=3
  Vb_hat : Inport  Port=4
  A_sens : Inport  Port=5
  Vned_hat : Inport  Port=6
  Demux : Demux  Outputs=3
  Embedded MATLAB Function1 : Stateflow chart
  "Get Roll, Pitch2" : Subsystem
  Integer Delay4 : simulink/Discrete/Integer Delay  vinit=0.0  samptime=-1  NumDelays=1
  Integer Delay5 : simulink/Discrete/Integer Delay  Orientation=left  vinit=0.0  samptime=-1  NumDelays=1
  Mux : Mux  Inputs=2
  Rate Transition{2,4..7} (5 alike) : RateTransition  OutPortSampleTime=T
  Sum5 : Sum  Inputs=|+-
  Sum6 : Sum  Inputs=-+|
  Sum7 : Sum  Inputs=-+|
  Terminator : Terminator
  get Centripetal : Subsystem
  Euler : Outport
  pqr_nb : Outport  Port=2
  wires:
  pqr_sens/1 -> Rate Transition2/1
  "b_{B}"/1 -> Rate Transition4/1
  Integer Delay4/1 -> Sum5/2
  Rate Transition6/1 -> Sum5/1
  Rate Transition4/1 -> Integer Delay4/1
  Vb_hat/1 -> Rate Transition5/1
  A_sens/1 -> Rate Transition6/1
  Rate Transition5/1 -> get Centripetal/2(Vb)
  Sum5/1 -> Sum6/2  "a"
  Sum6/1 -> "Get Roll, Pitch2"/1(Ab)  "a_mps"
  Rate Transition2/1 -> Sum7/2
  Sum7/1 -> get Centripetal/1(pqr), pqr_nb/1
  Vned_hat/1 -> Rate Transition7/1
  "Get Roll, Pitch2"/1("Phi, The") -> Mux/1
  "bg_{B}"/1 -> Integer Delay5/1
  Mux/1 -> Euler/1
  get Centripetal/1(w x Vb) -> Sum6/1
  Rate Transition7/1 -> Demux/1
  Demux/1 -> Embedded MATLAB Function1/1(Vn)
  Demux/2 -> Embedded MATLAB Function1/2(Ve)
  Embedded MATLAB Function1/1(cog) -> Mux/2
  Demux/3 -> Terminator/1

== system PositionComplementary/GPS Update/Detect Change ==
  Data : Inport
  Abs1 : Abs
  Difference1 : simulink/Discrete/Difference  SystemSampleTime=-1  ICPrevInput=0.0  OutDataType=sfix(16)  OutScaling=2^-10  DoSatur=off
  Saturation1 : Saturate  UpperLimit=1  LowerLimit=0  SampleTime=SampleT
  change? : Outport
  wires:
  Difference1/1 -> Abs1/1
  Abs1/1 -> Saturation1/1
  Data/1 -> Difference1/1
  Saturation1/1 -> change?/1

== system PositionComplementary/GPS Update/Detect Change1 ==
  Data : Inport
  Abs1 : Abs
  Difference1 : simulink/Discrete/Difference  SystemSampleTime=-1  ICPrevInput=0.0  OutDataType=sfix(16)  OutScaling=2^-10  DoSatur=off
  Saturation1 : Saturate  UpperLimit=1  LowerLimit=0  SampleTime=SampleT
  change? : Outport
  wires:
  Saturation1/1 -> change?/1
  Data/1 -> Difference1/1
  Abs1/1 -> Saturation1/1
  Difference1/1 -> Abs1/1

== system PositionComplementary/GPS Update/Detect Change2 ==
  Data : Inport
  Abs1 : Abs
  Difference1 : simulink/Discrete/Difference  SystemSampleTime=-1  ICPrevInput=0.0  OutDataType=sfix(16)  OutScaling=2^-10  DoSatur=off
  Saturation1 : Saturate  UpperLimit=1  LowerLimit=0  SampleTime=SampleT
  change? : Outport
  wires:
  Difference1/1 -> Abs1/1
  Abs1/1 -> Saturation1/1
  Data/1 -> Difference1/1
  Saturation1/1 -> change?/1

== system PositionComplementary/Get GPS in LTP/Geod2LTP2 ==
  "Height, Lat, Lon Initials from GPS" : Inport
  "Lat, deg(GPS)" : Inport  Port=2
  "Lon, deg(GPS)" : Inport  Port=3
  Hight,m(GPS) : Inport  Port=4
  Demux : Demux  Outputs=3
  ECEF2LTP (UEN) : Subsystem
      mask Display: plot(0,0,100,100,[45,40,35,40,40],[85,95,85,95,40],[85,95,85,95,40],[35,40,45,40,40],[60,40,10,20,10,14],[70,40,10,13,10,20],[56,45],[70,70],[60,60],[50,60],[60,60],[30,40],[50,60],[20,20],[30,40],[20,20],[45,55],[35,25],[75,65],[35,25])
  Geod2ECEF : Subsystem  mask{Re=6378137, Rp=6356752.3142}
      mask prompts: Re "Enter equatorial radius, m"; Rp "Enter polar radius,m"
  Geod2ECEF1 : Subsystem  mask{Re=6378137, Rp=6356752.3142}
      mask prompts: Re "Enter equatorial radius, m"; Rp "Enter polar radius,m"
  Mux : Mux  Inputs=3
  Mux1 : Mux  Inputs=2
  Mux2 : Mux  Inputs=3
  Reshape : Reshape  OutputDimensionality=Column vector (2-D)
  Sum1 : Sum  Inputs=|+-  SaturateOnIntegerOverflow=on
  UEN 2 NEU : Gain  Gain=[0 0 1;0 1 0;1 0 0]  Multiplication=Matrix(K*u)  SaturateOnIntegerOverflow=on
  "NEU, m" : Outport
  wires:
  UEN 2 NEU/1 -> "NEU, m"/1
  Geod2ECEF/3("Ze, m ") -> Mux/3
  Geod2ECEF/1("Xe, m ") -> Mux/1
  Geod2ECEF/2("Ye, m ") -> Mux/2
  "Lat, deg(GPS)"/1 -> Geod2ECEF/2("lat, deg")
  "Lon, deg(GPS)"/1 -> Geod2ECEF/3(lon,deg)
  Mux1/1 -> ECEF2LTP (UEN)/2("Long, Lat")
  Geod2ECEF1/3("Ze, m ") -> Mux2/3
  Geod2ECEF1/1("Xe, m ") -> Mux2/1
  Geod2ECEF1/2("Ye, m ") -> Mux2/2
  Mux2/1 -> Sum1/2  "R_in"
  Demux/1 -> Geod2ECEF1/1("height, m")
  Demux/2 -> Mux1/2, Geod2ECEF1/2("lat, deg")
  Demux/3 -> Mux1/1, Geod2ECEF1/3(lon,deg)
  ECEF2LTP (UEN)/1(Out) -> Reshape/1  "Moving Side"
  Hight,m(GPS)/1 -> Geod2ECEF/1("height, m")
  "Height, Lat, Lon Initials from GPS"/1 -> Demux/1
  Mux/1 -> Sum1/1  "r_mov"
  Sum1/1 -> ECEF2LTP (UEN)/1(ECEF coordinates)
  Reshape/1 -> UEN 2 NEU/1

== system PositionComplementary/Get GPS in LTP/Sim Latency ==
  Fast Data : Inport
  Counter Free-Running1 : simulink/Sources/Counter Free-Running  SystemSampleTime=-1  NumBits=1  tsamp=1
  Rate Transition2 : RateTransition  OutPortSampleTime=SampleT
  Sample and Hold : dspsigops/Sample and Hold  SystemSampleTime=-1  trig=Either edge  initCond=0  latchinput=off
  1Hz Data : Outport
  wires:
  Sample and Hold/1 -> 1Hz Data/1
  Fast Data/1 -> Sample and Hold/1
  Rate Transition2/1 -> Sample and Hold/Trigger
  Counter Free-Running1/1 -> Rate Transition2/1

== system PositionComplementary/Get GPS in LTP/Sim Latency3 ==
  Fast Data : Inport
  Counter Free-Running1 : simulink/Sources/Counter Free-Running  SystemSampleTime=-1  NumBits=1  tsamp=1
  Rate Transition2 : RateTransition  OutPortSampleTime=SampleT
  Sample and Hold : dspsigops/Sample and Hold  SystemSampleTime=-1  trig=Either edge  initCond=0  latchinput=off
  1Hz Data : Outport
  wires:
  Counter Free-Running1/1 -> Rate Transition2/1
  Rate Transition2/1 -> Sample and Hold/Trigger
  Fast Data/1 -> Sample and Hold/1
  Sample and Hold/1 -> 1Hz Data/1

== system PositionComplementary/Get GPS in LTP/Sim Latency4 ==
  Fast Data : Inport
  Counter Free-Running1 : simulink/Sources/Counter Free-Running  SystemSampleTime=-1  NumBits=1  tsamp=1
  Rate Transition2 : RateTransition  OutPortSampleTime=SampleT
  Sample and Hold : dspsigops/Sample and Hold  SystemSampleTime=-1  trig=Either edge  initCond=0  latchinput=off
  1Hz Data : Outport
  wires:
  Sample and Hold/1 -> 1Hz Data/1
  Fast Data/1 -> Sample and Hold/1
  Rate Transition2/1 -> Sample and Hold/Trigger
  Counter Free-Running1/1 -> Rate Transition2/1

== system PositionComplementary/Get GPS in LTP/Sim Latency5 ==
  Fast Data : Inport
  Counter Free-Running1 : simulink/Sources/Counter Free-Running  SystemSampleTime=-1  NumBits=1  tsamp=1
  Rate Transition2 : RateTransition  OutPortSampleTime=SampleT
  Sample and Hold : dspsigops/Sample and Hold  SystemSampleTime=-1  trig=Either edge  initCond=0  latchinput=off
  1Hz Data : Outport
  wires:
  Counter Free-Running1/1 -> Rate Transition2/1
  Rate Transition2/1 -> Sample and Hold/Trigger
  Fast Data/1 -> Sample and Hold/1
  Sample and Hold/1 -> 1Hz Data/1

== system PositionComplementary/Get GPS in LTP/Sim Latency6 ==
  Fast Data : Inport
  Counter Free-Running1 : simulink/Sources/Counter Free-Running  SystemSampleTime=-1  NumBits=1  tsamp=1
  Rate Transition2 : RateTransition  OutPortSampleTime=SampleT
  Sample and Hold : dspsigops/Sample and Hold  SystemSampleTime=-1  trig=Either edge  initCond=0  latchinput=off
  1Hz Data : Outport
  wires:
  Sample and Hold/1 -> 1Hz Data/1
  Fast Data/1 -> Sample and Hold/1
  Rate Transition2/1 -> Sample and Hold/Trigger
  Counter Free-Running1/1 -> Rate Transition2/1

== system PositionComplementary/Plant Model/Plant ==
  de : Inport
  da : Inport  Port=2
  dr : Inport  Port=3
  dt : Inport  Port=4
  df : Inport  Port=5
  6-DOF EOM : Subsystem
  Engine Model : Subsystem
  Forces and Moments : Subsystem
  Get GPS : Subsystem
  ISA Atmosphere & Winds : Subsystem  Orientation=left
  Mux : Mux  Inputs=2
  Scope : Scope
      settings: YMin=0  YMax=5250
  Sum : Sum  Inputs=++|  SaturateOnIntegerOverflow=on
  GPS Month : Outport
  GPS Day : Outport  Port=2
  GPS Year : Outport  Port=3
  GPS Hr : Outport  Port=4
  GPS Min : Outport  Port=5
  GPS Sec : Outport  Port=6
  GPS Frac Sec : Outport  Port=7
  GPS Lat (rad) : Outport  Port=8
  GPS Long (rad) : Outport  Port=9
  GPS H (m) : Outport  Port=10
  PQR : Outport  Port=11
  Ab : Outport  Port=12
  Dynamic : Outport  Port=13
  Static : Outport  Orientation=left  Port=14
  Euler : Outport  Port=15
  Vmag : Outport  Port=16
  RPM : Outport  Port=17
  Vned : Outport  Port=18
  aoa/betta,deg : Outport  Port=19
  Ab meas : Outport  Port=20
  Vb : Outport  Port=21
  Euler_dot : Outport  Port=22
  wires:
  Get GPS/1(GPS Month) -> GPS Month/1
  Get GPS/2(GPS Day) -> GPS Day/1
  Get GPS/3(GPS Year) -> GPS Year/1
  Get GPS/4(GPS Hr) -> GPS Hr/1
  Get GPS/5(GPS Min) -> GPS Min/1
  Get GPS/6(GPS Sec) -> GPS Sec/1
  Get GPS/7(GPS Frac Sec) -> GPS Frac Sec/1
  Get GPS/8(GPS Lat (rad)) -> GPS Lat (rad)/1
  Get GPS/9(GPS Long (rad)) -> GPS Long (rad)/1
  Get GPS/10(GPS H (m)) -> GPS H (m)/1
  6-DOF EOM/8(Ab meas) -> Ab meas/1
  Mux/1 -> 6-DOF EOM/1("[F,M]")
  6-DOF EOM/5(Euler_dot) -> Euler_dot/1
  6-DOF EOM/6(Vb) -> Vb/1
  Engine Model/1(RPM) -> RPM/1
  Engine Model/2(Thrust) -> Sum/1
  Forces and Moments/6(q) -> Dynamic/1
  ISA Atmosphere & Winds/3(AirPressure (Pa)) -> Static/1
  Forces and Moments/1(Airspeed) -> Engine Model/2(Vmag), Vmag/1
  ISA Atmosphere & Winds/2(Wind) -> Forces and Moments/1(Wind e)
  ISA Atmosphere & Winds/1(Rho) -> Forces and Moments/2(Rho)
  Forces and Moments/3(Moments) -> Mux/2
  Forces and Moments/2(Forces) -> Sum/2
  Sum/1 -> Mux/1
  Forces and Moments/4(Vb Corr) -> 6-DOF EOM/2(Vb Corr)
  6-DOF EOM/1(X,Y,Z (LTP)) -> ISA Atmosphere & Winds/1("X, Y, Z"), Get GPS/1(XYZ (NEU)), Scope/1  "position"
  6-DOF EOM/2("Vx, Vy, Vz") -> Vned/1, Forces and Moments/7("Vx, Vy, Vz ")  "velocity"
  6-DOF EOM/3(Euler) -> Forces and Moments/8(Euler), Euler/1  "Euler angles"
  6-DOF EOM/4("p, q, r") -> PQR/1, Forces and Moments/9(p,q,r)  "rates"
  6-DOF EOM/7(Ab) -> Ab/1
  Forces and Moments/5("aoa/betta, deg") -> aoa/betta,deg/1
  dt/1 -> Engine Model/1(dt)
  de/1 -> Forces and Moments/3("de, deg")
  da/1 -> Forces and Moments/4(da,deg)
  dr/1 -> Forces and Moments/5("dr, deg")
  df/1 -> Forces and Moments/6("df, deg")

== system PositionComplementary/Position  Complementary Filter/Subsystem ==
  Euler_hat : Inport  Orientation=left
  Integer Delay2 : simulink/Discrete/Integer Delay  Orientation=left  vinit=0.0  samptime=-1  NumDelays=1
  LTP2B : dspmtrx3/Transpose  Orientation=left  SystemSampleTime=-1  Hermitian=off  overflowFlag=off
  RB2LTP : Subsystem  Orientation=left
  RB2LT : Outport  Orientation=left
  RLT2B : Outport  Orientation=left  Port=2
  wires:
  RB2LTP/1(Rot) -> RB2LT/1, LTP2B/1
  LTP2B/1 -> RLT2B/1
  Integer Delay2/1 -> RB2LTP/1(Euler)
  Euler_hat/1 -> Integer Delay2/1

== system PositionComplementary/Signal Cond/Accel Convert ==
  Raw : Inport
  3vector LPF : Subsystem  mask{flpf=5}
      mask prompts: flpf "LowPass Freq"
      mask Display: droots([],-flpf,flpf)
  Bias : Constant  Value=[2015 2018 2006]
  Divide : Product  Inputs=/*  OutScaling=2^-10
  Gains : Constant  Value=[-41 41 -43]
  Scope2 : Scope
      settings: TimeRange=100  YMin=-14.06123404388128  YMax=1.094597546893038  SaveName=ScopeData25
  Sum : Sum  Inputs=|+-
  Comp : Outport
  wires:
  Raw/1 -> 3vector LPF/1(In1)
  Divide/1 -> Comp/1, Scope2/1
  Sum/1 -> Divide/2
  Gains/1 -> Divide/1
  Bias/1 -> Sum/2
  3vector LPF/1(Out1) -> Sum/1

== system PositionComplementary/Signal Cond/Gyro Convert ==
  Raw : Inport
  3vector LPF : Subsystem  mask{flpf=5}
      mask prompts: flpf "LowPass Freq"
      mask Display: droots([],-flpf,flpf)
  Bias : Constant  Value=[1866 1981 2042]
  Divide : Product  Inputs=/*  OutScaling=2^-10
  Gains : Constant  Value=[-142 142 235]
  Sum : Sum  Inputs=|+-
  Comp : Outport
  wires:
  Bias/1 -> Sum/2
  Gains/1 -> Divide/1
  Sum/1 -> Divide/2
  Divide/1 -> Comp/1
  Raw/1 -> 3vector LPF/1(In1)
  3vector LPF/1(Out1) -> Sum/1

== system PositionComplementary/Subsystem3/Autopilot ==
  Sensors : Inport  PortDimensions=SizeSensors
  Estimates : Inport  Port=2  PortDimensions=SizeEstim
  Settings : Inport  Port=3  PortDimensions=SizeSet
  Commands : Inport  Port=4  PortDimensions=SizeCmd
  States : Inport  Port=5  PortDimensions=SizeStates
  Gains : Inport  Port=6  PortDimensions=SizeGains
  Limits : Inport  Port=7  PortDimensions=SizeLimits
  Autopilot Enable : EnablePort  StatesWhenEnabling=reset
  Air System Vector Inputs : piccolo_library/Flight Mechanics/Air System Vector Inputs  SystemSampleTime=-1  tsamp=APtsamp
  Altitude Control Vector Inputs : Subsystem  AncestorBlock=piccolo_library/Controllers/Longitudinal/Altitude Control Vector Inputs
  Demux{,1..6} (7 alike) : Demux  Outputs=7
  Flap Control Vector Inputs : Subsystem
  Gain : Gain  SaturateOnIntegerOverflow=on
  Gain1 : Gain  SaturateOnIntegerOverflow=on
  Guidance & Navigation Vector Input : Subsystem  AncestorBlock=piccolo_library/Controllers/Guidance/Guidance & Navigation Vector Input
  Mux : Mux  Inputs=12
  Mux1 : Mux  Inputs=5
  Mux2 : Mux  Inputs=7
  Pitch Control  Vector Inputs : Subsystem  AncestorBlock="piccolo_library/Controllers/Longitudinal/Pitch Control  Vector Inputs"
  Reserved Outputs : Constant  Value=0
  Roll Control Vector Inputs : Subsystem  AncestorBlock=piccolo_library/Controllers/Lateral/Roll Control Vector Inputs
  Yaw Control Vector Inputs : Subsystem  AncestorBlock=piccolo_library/Controllers/Lateral/Yaw Control Vector Inputs
  Actuators : Outport  OutDataType=fixdt(1,16,0)  OutScaling=[]
  Derived : Outport  Port=2  OutDataType=fixdt(1,16,0)  OutScaling=[]
  NPSTrim : Outport  Port=3  OutDataType=fixdt(1,16,0)  OutScaling=[]
  wires:
  Mux/1 -> Gain/1, NPSTrim/1
  Mux1/1 -> Roll Control Vector Inputs/8(Derived), Altitude Control Vector Inputs/8(Derived), Pitch Control  Vector Inputs/8(Derived), Guidance & Navigation Vector Input/8(Derived), Yaw Control Vector Inputs/8(Derived), Air System Vector Inputs/8, Flap Control Vector Inputs/8(Derived), Gain1/1
  Roll Control Vector Inputs/1(Actuator) -> Mux/2
  Pitch Control  Vector Inputs/1(Actuator) -> Mux/4
  Altitude Control Vector Inputs/1(Actuator) -> Mux/8
  Sensors/1 -> Mux2/1
  Estimates/1 -> Mux2/2
  Settings/1 -> Mux2/3
  Commands/1 -> Mux2/4
  States/1 -> Mux2/5
  Gains/1 -> Mux2/6
  Limits/1 -> Mux2/7
  Demux/1 -> Altitude Control Vector Inputs/1(Sensors)
  Demux/2 -> Altitude Control Vector Inputs/2(Estimates)
  Demux/3 -> Altitude Control Vector Inputs/3(Settings)
  Demux/4 -> Altitude Control Vector Inputs/4(Commands)
  Demux/5 -> Altitude Control Vector Inputs/5(States)
  Demux/6 -> Altitude Control Vector Inputs/6(Gains)
  Demux/7 -> Altitude Control Vector Inputs/7(Limits)
  Demux1/1 -> Roll Control Vector Inputs/1(Sensors)
  Demux1/2 -> Roll Control Vector Inputs/2(Estimates)
  Demux1/3 -> Roll Control Vector Inputs/3(Settings)
  Demux1/4 -> Roll Control Vector Inputs/4(Commands)
  Demux1/5 -> Roll Control Vector Inputs/5(States)
  Demux1/6 -> Roll Control Vector Inputs/6(Gains)
  Demux1/7 -> Roll Control Vector Inputs/7(Limits)
  Demux2/1 -> Pitch Control  Vector Inputs/1(Sensors)
  Demux2/2 -> Pitch Control  Vector Inputs/2(Estimates)
  Demux2/3 -> Pitch Control  Vector Inputs/3(Settings)
  Demux2/4 -> Pitch Control  Vector Inputs/4(Commands)
  Demux2/5 -> Pitch Control  Vector Inputs/5(States)
  Demux2/6 -> Pitch Control  Vector Inputs/6(Gains)
  Demux2/7 -> Pitch Control  Vector Inputs/7(Limits)
  Demux3/1 -> Guidance & Navigation Vector Input/1(Sensors)
  Demux3/2 -> Guidance & Navigation Vector Input/2(Estimates)
  Demux3/3 -> Guidance & Navigation Vector Input/3(Settings)
  Demux3/4 -> Guidance & Navigation Vector Input/4(Commands)
  Demux3/5 -> Guidance & Navigation Vector Input/5(States)
  Demux3/6 -> Guidance & Navigation Vector Input/6(Gains)
  Demux3/7 -> Guidance & Navigation Vector Input/7(Limits)
  Demux4/1 -> Yaw Control Vector Inputs/1(Sensors)
  Demux4/2 -> Yaw Control Vector Inputs/2(Estimates)
  Demux4/3 -> Yaw Control Vector Inputs/3(Settings)
  Demux4/4 -> Yaw Control Vector Inputs/4(Commands)
  Demux4/5 -> Yaw Control Vector Inputs/5(States)
  Demux4/6 -> Yaw Control Vector Inputs/6(Gains)
  Demux4/7 -> Yaw Control Vector Inputs/7(Limits)
  Demux5/1 -> Air System Vector Inputs/1
  Demux5/2 -> Air System Vector Inputs/2
  Demux5/3 -> Air System Vector Inputs/3
  Demux5/4 -> Air System Vector Inputs/4
  Demux5/5 -> Air System Vector Inputs/5
  Demux5/6 -> Air System Vector Inputs/6
  Demux5/7 -> Air System Vector Inputs/7
  Mux2/1 -> Demux1/1, Demux/1, Demux2/1, Demux3/1, Demux4/1, Demux5/1, Demux6/1
  Reserved Outputs/1 -> Mux/11, Mux/9, Mux/7, Mux/1, Mux/3, Mux/5, Mux/12
  Yaw Control Vector Inputs/1(Actuator) -> Mux/6
  Flap Control Vector Inputs/1(Actuator) -> Mux/10
  Demux6/1 -> Flap Control Vector Inputs/1(Sensors)
  Demux6/2 -> Flap Control Vector Inputs/2(Estimates)
  Demux6/3 -> Flap Control Vector Inputs/3(Settings)
  Demux6/4 -> Flap Control Vector Inputs/4(Commands)
  Demux6/5 -> Flap Control Vector Inputs/5(States)
  Demux6/6 -> Flap Control Vector Inputs/6(Gains)
  Demux6/7 -> Flap Control Vector Inputs/7(Limits)
  Air System Vector Inputs/1 -> Mux1/1
  Roll Control Vector Inputs/2(Param) -> Mux1/2
  Pitch Control  Vector Inputs/2(Param) -> Mux1/3
  Guidance & Navigation Vector Input/1(Param) -> Mux1/4
  Altitude Control Vector Inputs/2(Param) -> Mux1/5
  Gain/1 -> Actuators/1
  Gain1/1 -> Derived/1
